simulink model "vrpinvex"  (Simulink 3.00)
settings: Solver=FixedStepDiscrete  StartTime=0.0  StopTime=499  RelTol=1e-3
libraries: smxl x4, simulink3 x1
settings Model: LastModifiedBy=giampiero

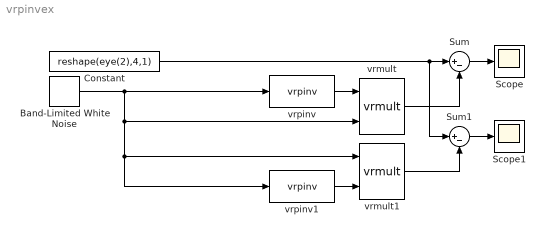
== system vrpinvex ==
  Band-Limited White Noise : simulink3/Sources/Band-Limited White Noise  Cov=[0.1]*ones(6,1)  Ts=0.1  seed=1:6
  Constant : Constant  Value=reshape(eye(2),4,1)
  Scope : Scope
      settings: TimeRange=500  YMin=-4e-015  YMax=4e-015  SaveToWorkspace=off  SaveName=ScopeData
  Scope1 : Scope
      settings: TimeRange=500  YMin=-4e-015  YMax=4e-015  SaveToWorkspace=off  SaveName=ScopeData
  Sum : Sum  Inputs=|+-  SaturateOnIntegerOverflow=on
  Sum1 : Sum  Inputs=|+-  SaturateOnIntegerOverflow=on
  vrmult : smxl/Real Matrices/vrmult  dims=[2 3 2]
  vrmult1 : smxl/Real Matrices/vrmult  dims=[2 3 2]
  vrpinv : smxl/Real Matrices/vrpinv  dims=[3 2]  tol=1
  vrpinv1 : smxl/Real Matrices/vrpinv  dims=[2 3]  tol=1
  wires:
  Band-Limited White Noise/1 -> vrpinv/1, vrmult/2, vrmult1/1, vrpinv1/1
  vrpinv/1 -> vrmult/1
  Sum/1 -> Scope/1
  vrmult1/1 -> Sum1/2
  Sum1/1 -> Scope1/1
  vrmult/1 -> Sum/2
  Constant/1 -> Sum/1, Sum1/1
  vrpinv1/1 -> vrmult1/2
